simulink model "iface2"  (R2018b)
settings: Solver=FixedStepDiscrete  StartTime=0.0  StopTime=10.0  RelTol=1e-3
undefined symbols (not defined in the file): myBool, myInteger, myReal, mySeqOfVar
settings Model: Creator=matlab  LastModifiedBy=matlab
settings DataIOCC: SaveOutput=off  SignalLogging=off  SaveTime=off
settings OptimizationCC: DefaultParameterBehavior=Inlined  EnhancedBackFolding=on  PassReuseOutputArgsAs=Individual arguments  OptimizeBlockOrder=speed  DifferentSizesBufferReuse=on  OptimizationCustomize=off
settings DebuggingCC: ParameterTunabilityLossMsg=error
settings SFSimCC: MATLABDynamicMemAlloc=off
settings RTWCC: SystemTargetFile=ert.tlc  TemplateMakefile=ert_default_tmf  PostCodeGenCommand=packNGo(buildInfo);  GenerateReport=on  IncludeHyperlinkInReport=on  LaunchReport=on  GenerateTraceInfo=on  GenerateTraceReport=on  GenerateTraceReportSl=on  GenerateTraceReportSf=on  GenerateTraceReportEml=on
settings CodeAppCC: ForceParamTrailComments=on  IgnoreCustomStorageClasses=off  OperatorAnnotations=on  SimulinkDataObjDesc=on  SFDataObjDesc=on  InsertBlockDesc=on
settings ERTTargetCC: TargetLangStandard=C99 (ISO)  GenerateSampleERTMain=on  InlinedParameterPlacement=NonHierarchical  ERTCustomFileTemplate=example_file_process.tlc

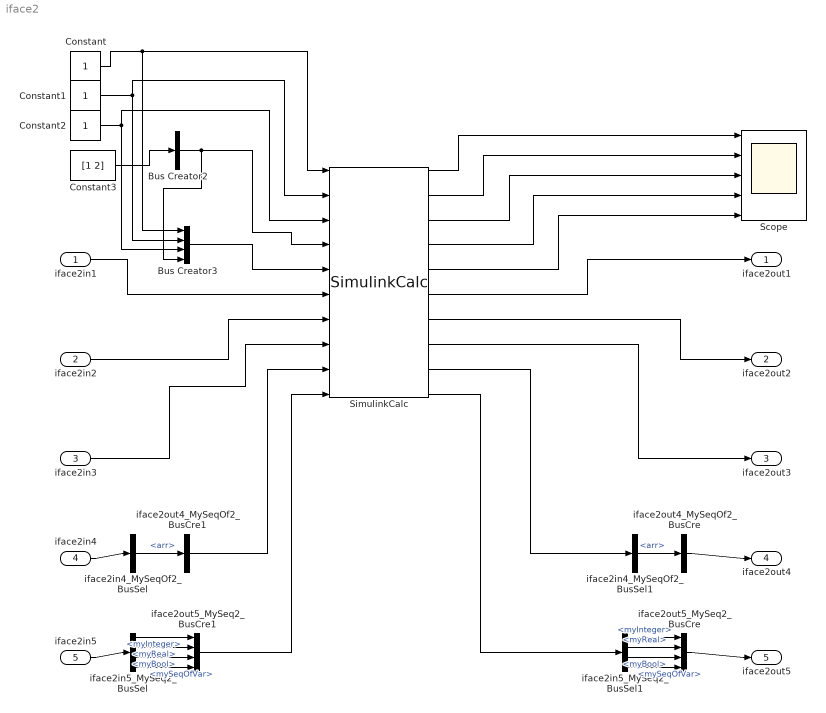
== system iface2 ==
  iface2in1 : Inport  OutDataTypeStr=MyInteger2  BusOutputAsStruct=on
  iface2in2 : Inport  Port=2  OutDataTypeStr=MyReal2  BusOutputAsStruct=on
  iface2in3 : Inport  Port=3  OutDataTypeStr=MyBool2  BusOutputAsStruct=on
  iface2in4 : Inport  Port=4  OutDataTypeStr=Bus: MySeqOf2  BusOutputAsStruct=on
  iface2in5 : Inport  Port=5  OutDataTypeStr=Bus: MySeq2  BusOutputAsStruct=on
  Bus Creator2 : BusCreator  Inputs=1  OutDataTypeStr=Bus: MySeqOf  NonVirtualBus=on
  Bus Creator3 : BusCreator  Inputs=4  OutDataTypeStr=Bus: MySeq  NonVirtualBus=on
  Constant : Constant  OutDataTypeStr=MyInteger
  Constant1 : Constant  OutDataTypeStr=MyReal
  Constant2 : Constant  OutDataTypeStr=MyBool
  Constant3 : Constant  Value=[1 2]  OutDataTypeStr=MyInteger
  Scope : Scope  NumInputPorts=5
  SimulinkCalc : S-Function  FunctionName=SimulinkCalc  SFunctionDeploymentMode=off  EnableBusSupport=off  mask(Legacy Function){SFunctionSpec=void simulink_RI_calc(MyInteger u1[1], MyReal u2[1], MyBool u3[1], MySeqOf u4[1], MySeq u5[1], MyInteger y1[1], MyReal y2[1], MyBool y3[1], MySeqOf y4[1], MySeq y5[1], MyInteger2 u6[1], MyReal2 u7[1], MyBool2 u8[1], MySeqOf2 u9[1], MySeq2 u10[1], MyInteger2 y6[1], MyReal2 y7[1], MyBool2 y8[1], MySeqOf2 y9[1], MySeq2 y10[1]), ShowSpec=off}
      mask prompts: ShowSpec "Display function specification"
      mask help:
      | This block allows you to call the legacy functions specified by the following Legacy Code Tool definition:
      | def.SFunctionName = 'SimulinkCalc';
      | def.OutputFcnSpec = 'void simulink_RI_calc(MyInteger u1[1], MyReal u2[1], MyBool u3[1], MySeqOf u4[1], MySeq u5[1], MyInteger y1[1], MyReal y2[1], MyBool y3[1], MySeqOf y4[1], MySeq y5[1], MyInteger2 u6[1], MyReal2 u7[1], MyBool2 u8[1], MySeqOf2 u9[1], MySeq2 u10[1], MyInteger2 y6[1], MyReal2 y7[1], MyBool2 y8[1], MySeqOf2 y9[1], MySeq2 y10[1])';
      | def.HeaderFiles = {'simulink_invoke_ri.h'};
      | def.SourceFiles = {'simulink_invoke_ri.c'};
      | def.IncPaths = {'..\..\..\dataview\C'};
      mask Help: <p>This block was generated automatically by the Legacy Code Tool. For detailed help on this tool, call<a href="matlab:legacy_code('help')"> legacy_code('help')</a>.</p>
      mask Callback ShowSpec:
      | if strcmp(get_param(gcbh, 'ShowSpec'), 'on')
      |   set_param(gcbh, 'MaskDisplay', sprintf('fprintf(''%s'');', get_param(gcbh, 'SFunctionSpec')));
      | else
      |   set_param(gcbh, 'MaskDisplay', sprintf('fprintf(''%s'');', get_param(gcbh, 'FunctionName')));
      | end
      mask Display: fprintf('SimulinkCalc');
  iface2in4_MySeqOf2_BusSel : BusSelector  OutputSignals=arr
  iface2in4_MySeqOf2_BusSel1 : BusSelector  OutputSignals=arr
  iface2in5_MySeq2_BusSel : BusSelector  OutputSignals=myInteger,myReal,myBool,mySeqOfVar
  iface2in5_MySeq2_BusSel1 : BusSelector  OutputSignals=myInteger,myReal,myBool,mySeqOfVar
  iface2out4_MySeqOf2_BusCre : BusCreator  Inputs=1  OutDataTypeStr=Bus: MySeqOf2  NonVirtualBus=on
  iface2out4_MySeqOf2_BusCre1 : BusCreator  Inputs=1  OutDataTypeStr=Bus: MySeqOf2  NonVirtualBus=on
  iface2out5_MySeq2_BusCre : BusCreator  Inputs=myInteger,myReal,myBool,mySeqOfVar  OutDataTypeStr=Bus: MySeq2  NonVirtualBus=on
  iface2out5_MySeq2_BusCre1 : BusCreator  Inputs=myInteger,myReal,myBool,mySeqOfVar  OutDataTypeStr=Bus: MySeq2  NonVirtualBus=on
  iface2out1 : Outport  OutDataTypeStr=MyInteger2
  iface2out2 : Outport  Port=2  OutDataTypeStr=MyReal2
  iface2out3 : Outport  Port=3  OutDataTypeStr=MyBool2
  iface2out4 : Outport  Port=4  OutDataTypeStr=Bus: MySeqOf2  BusOutputAsStruct=on
  iface2out5 : Outport  Port=5  OutDataTypeStr=Bus: MySeq2  BusOutputAsStruct=on
  wires:
  iface2in4/1 -> iface2in4_MySeqOf2_BusSel/1
  iface2in5/1 -> iface2in5_MySeq2_BusSel/1
  iface2out4_MySeqOf2_BusCre/1 -> iface2out4/1
  iface2out5_MySeq2_BusCre/1 -> iface2out5/1
  Constant3/1 -> Bus Creator2/1
  Constant/1 -> SimulinkCalc/1, Bus Creator3/1
  Bus Creator2/1 -> SimulinkCalc/4, Bus Creator3/4
  Constant1/1 -> SimulinkCalc/2, Bus Creator3/2
  Constant2/1 -> SimulinkCalc/3, Bus Creator3/3
  Bus Creator3/1 -> SimulinkCalc/5
  iface2in1/1 -> SimulinkCalc/6
  iface2in2/1 -> SimulinkCalc/7
  iface2in3/1 -> SimulinkCalc/8
  iface2out5_MySeq2_BusCre1/1 -> SimulinkCalc/10
  iface2out4_MySeqOf2_BusCre1/1 -> SimulinkCalc/9
  iface2in4_MySeqOf2_BusSel/1 -> iface2out4_MySeqOf2_BusCre1/1  "<arr>"
  iface2in5_MySeq2_BusSel/1 -> iface2out5_MySeq2_BusCre1/1  "<myInteger>"
  iface2in5_MySeq2_BusSel/2 -> iface2out5_MySeq2_BusCre1/2  "<myReal>"
  iface2in5_MySeq2_BusSel/3 -> iface2out5_MySeq2_BusCre1/3  "<myBool>"
  iface2in5_MySeq2_BusSel/4 -> iface2out5_MySeq2_BusCre1/4  "<mySeqOfVar>"
  iface2in5_MySeq2_BusSel1/2 -> iface2out5_MySeq2_BusCre/2  "<myReal>"
  iface2in5_MySeq2_BusSel1/3 -> iface2out5_MySeq2_BusCre/3  "<myBool>"
  iface2in4_MySeqOf2_BusSel1/1 -> iface2out4_MySeqOf2_BusCre/1  "<arr>"
  SimulinkCalc/10 -> iface2in5_MySeq2_BusSel1/1
  iface2in5_MySeq2_BusSel1/4 -> iface2out5_MySeq2_BusCre/4  "<mySeqOfVar>"
  iface2in5_MySeq2_BusSel1/1 -> iface2out5_MySeq2_BusCre/1  "<myInteger>"
  SimulinkCalc/9 -> iface2in4_MySeqOf2_BusSel1/1
  SimulinkCalc/8 -> iface2out3/1
  SimulinkCalc/7 -> iface2out2/1
  SimulinkCalc/6 -> iface2out1/1
  SimulinkCalc/1 -> Scope/1
  SimulinkCalc/2 -> Scope/2
  SimulinkCalc/3 -> Scope/3
  SimulinkCalc/4 -> Scope/4
  SimulinkCalc/5 -> Scope/5
